simulink library "ecef_2_TLE_lib"  (R2016b)
settings: Solver=VariableStepAuto  StartTime=0.0  StopTime=10.0  RelTol=1e-3
undefined symbols (not defined in the file or in its folder): fsw_params
libraries: ECI2OEV_lib x1, time_coord_rotation_lib x1
settings Model: Creator=taylorreynolds  LastModifiedBy=taylorreynolds

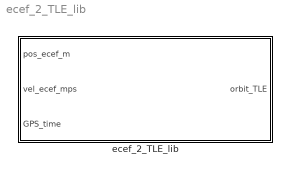
== system ecef_2_TLE_lib ==
  ecef_2_TLE_lib : Subsystem

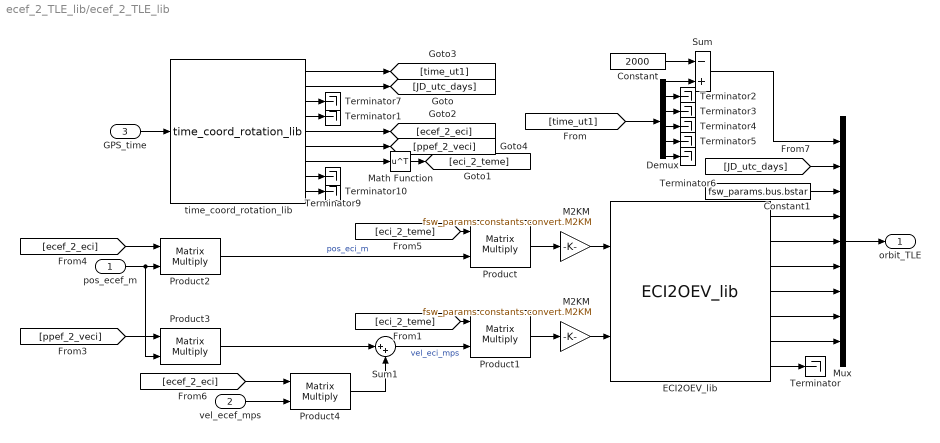
== system ecef_2_TLE_lib/ecef_2_TLE_lib ==
  pos_ecef_m : Inport
  vel_ecef_mps : Inport  Port=2
  GPS_time : Inport  Port=3
  Constant : Constant  Value=2000
  Constant1 : Constant  Value=fsw_params.bus.bstar
  Demux : Demux  Outputs=6
  ECI2OEV_lib : ECI2OEV_lib/ECI2OEV_lib
  M2KM : Gain  Gain=fsw_params.constants.convert.M2KM
  "M2KM " : Gain  Gain=fsw_params.constants.convert.M2KM
  Math Function : Math  Operator=transpose  SaturateOnIntegerOverflow=on
  Mux : Mux  Inputs=9
  Product{,1..4} (5 alike) : Product  Multiplication=Matrix(*)
  Sum : Sum  Inputs=-+
  Sum1 : Sum  Inputs=|++
  Terminator{,1..7,9..10} (10 alike) : Terminator
  time_coord_rotation_lib : time_coord_rotation_lib/time_coord_rotation_lib
  orbit_TLE : Outport
  wires:
  GPS_time/1 -> time_coord_rotation_lib/1
  [JD_utc_days] -> Mux/2
  vel_ecef_mps/1 -> Product4/2
  pos_ecef_m/1 -> Product3/2, Product2/2
  Constant1/1 -> Mux/3
  Demux/6 -> Terminator6/1
  Demux/5 -> Terminator5/1
  Demux/4 -> Terminator4/1
  Demux/3 -> Terminator3/1
  Demux/2 -> Terminator2/1
  Demux/1 -> Sum/2
  Sum/1 -> Mux/1
  Constant/1 -> Sum/1
  [time_ut1] -> Demux/1
  Mux/1 -> orbit_TLE/1
  M2KM/1 -> ECI2OEV_lib/1
  "M2KM "/1 -> ECI2OEV_lib/2
  ECI2OEV_lib/1 -> Mux/4
  ECI2OEV_lib/2 -> Mux/5
  ECI2OEV_lib/3 -> Mux/6
  ECI2OEV_lib/4 -> Mux/7
  ECI2OEV_lib/5 -> Mux/8
  ECI2OEV_lib/6 -> Mux/9
  Product/1 -> M2KM/1
  Product1/1 -> "M2KM "/1
  [ecef_2_eci] -> Product2/1
  Product2/1 -> Product/2  "pos_eci_m"
  Math Function/1 -> [eci_2_teme]
  [eci_2_teme] -> Product/1
  [eci_2_teme] -> Product1/1
  Product3/1 -> Sum1/1
  [ppef_2_veci] -> Product3/1
  [ecef_2_eci] -> Product4/1
  Product4/1 -> Sum1/2
  Sum1/1 -> Product1/2  "vel_eci_mps"
  time_coord_rotation_lib/9 -> Terminator10/1
  time_coord_rotation_lib/8 -> Terminator9/1
  time_coord_rotation_lib/7 -> Math Function/1
  time_coord_rotation_lib/6 -> [ppef_2_veci]
  time_coord_rotation_lib/1 -> [time_ut1]
  time_coord_rotation_lib/3 -> Terminator7/1
  time_coord_rotation_lib/4 -> Terminator1/1
  time_coord_rotation_lib/5 -> [ecef_2_eci]
  time_coord_rotation_lib/2 -> [JD_utc_days]
  ECI2OEV_lib/7 -> Terminator/1
